simulink model "q_bb01_pos"  (R2021b)
settings: Solver=ode4  StartTime=0.0  StopTime=inf  FixedStep=0.002  RelTol=1e-3  AbsTol=1e-6  EnableMultiTasking=on
values from neighbouring files (symbols this model uses):
  K_AMP = 1    [setup_srv02_exp04_bb01.m]
  K_BS = - L_beam / 10    [config_bb01.m]    (also in setup_srv02_exp04_bb01.m = 2 * K_BS)
  Kc = wn^2 / (Tp*K_bb*z*wf)    [d_bb01_pd.m]    (also in setup_srv02_exp04_bb01.m = 0)
  kp = (wn^2/K)*tau    [d_pv_design.m]    (also in setup_srv02_exp04_bb01.m = 0)
  kv = (-1+2*zeta*wn*tau)/K    [d_pv_design.m]    (also in setup_srv02_exp04_bb01.m = 0)
  THETA_MAX = 56.0 * K_D2R    [config_bb01.m]
  THETA_MIN = - 56.0 * K_D2R    [config_bb01.m]
  THETA_OFF = - 56.0 * K_D2R    [config_bb01.m]
  VMAX_DAC = 10    [setup_srv02_exp04_bb01.m]
  wcf = 2 * pi * 50.0    (= 314.159265359)    [setup_srv02_exp04_bb01.m]
  wf = 2 * pi * 2.5    (= 15.7079632679)    [d_bb01_pd.m]    (also in setup_srv02_exp04_bb01.m = 6.28318530718)
  z = wn*wf/(-wn+wf*wn*Tp+2*wf*zeta)    [d_bb01_pd.m]    (also in setup_srv02_exp04_bb01.m = 1)
  zetaf = 0.9    [setup_srv02_exp04_bb01.m]
undefined symbols (not defined in the file or in its folder): HIL, K_ENC, qc_get_step_size, VMAX_AMP
libraries: simulink x6, quarc_library x6, simulink_extras x1
settings Model: SimulationMode=external  ExtModeTrigDuration=25000  Creator=MLevis  LastModifiedBy=Dell
settings SolverCC: AutoScaleAbsTol=off  AlgebraicLoopSolver=TrustRegion  PositivePriorityOrder=on
settings DataIOCC: SaveFormat=Array  SignalLoggingSaveFormat=ModelDataLogs  ReturnWorkspaceOutputs=off
settings OptimizationCC: BlockReduction=off  BooleanDataType=off  OptimizeBlockIOStorage=off  BufferReuse=off  ExpressionFolding=off  ExpressionDepthLimit=2147483647  LocalBlockOutputs=off  InitFltsAndDblsToZero=on
settings DebuggingCC: SaveWithParameterizedLinksMsg=none  UnderspecifiedInitializationDetection=Classic  MergeDetectMultiDrivingBlocksExec=none  SignalResolutionControl=TryResolveAllWithWarning  MultiTaskDSMMsg=warning  MultiTaskCondExecSysMsg=none  FcnCallInpInsideContextMsg=warning  StateNameClashWarn=warning  SFUnexpectedBacktrackingDiag=warning  SFNoUnconditionalDefaultTransitionDiag=warning  SFExecutionAtInitializationDiag=none  SFMachineParentedDataDiag=warning  ArithmeticOperatorsInVariantConditions=warning
settings HardwareCC: TargetHWDeviceType=32-bit Generic
settings ModelReferenceCC: PropagateSignalLabelsOutOfModel=off
settings RTWCC: Description=QUARC Win64 Target Using Toolchain  SystemTargetFile=quarc_win64.tlc  TemplateMakefile=quarc_default_tmf  Toolchain=QUARC win64 | nmake (64-bit Windows)  BuildConfiguration=Faster Runs
settings CodeAppCC: StateflowObjectComments=on
settings STFCustomTargetCC: ConcurrentExecutionCompliant=on  UseToolchainInfoCompliant=on  SystemTargetFile=quarc_win64.tlc
settings GRTTargetCC: TargetLangStandard=C89/C90 (ANSI)  ParMdlRefBuildCompliant=off  CompOptLevelCompliant=off  CombineOutputUpdateFcns=off  MatFileLogging=off  CPPClassGenCompliant=off  GRTInterface=on  ExtMode=on  ExtModeMexFile=quarc_comm
settings ConfigComp: CovMetricSettings=dw  CovSaveCumulativeToWorkspaceVar=on  CovSaveSingleToWorkspaceVar=on

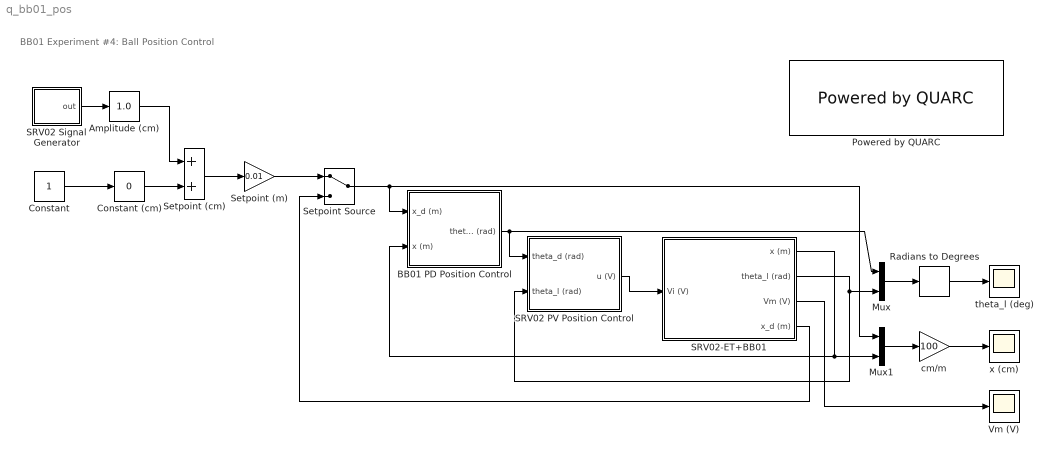
== system q_bb01_pos ==
  note: BB01 Experiment #4: Ball Position Control
  Amplitude (cm) : simulink/Math Operations/Slider Gain  gain=1.0  low=-10  high=10
  BB01 PD Position Control : Subsystem
  "Constant " : Constant
  Constant (cm) : simulink/Math Operations/Slider Gain  gain=0  low=-20  high=20
  Mux : Mux  Inputs=2
  Mux1 : Mux  Inputs=2
  Powered by QUARC : quarc_library/Logos/Powered by QUARC
  Radians to Degrees : simulink_extras/Transformations/Radians to Degrees
  SRV02 PV Position Control : Subsystem
  SRV02 Signal Generator : Subsystem  mask(QET Signal Generator){sig_type=square, a=2, f=0.4}
      mask prompts: sig_type "Signal Type"; a "Amplitude"; f "Frequency (Hz)"
      mask help: Generates a square, triangular, or sinusoidal waveform of a specified amplitude and frequency.
      mask Help: Choose the type of signal to be generated from the drop-down "Signal Type" box. Enter the amplitude and the frequency desired for the signal. Note: frequency is in Hertz.
      mask TypeOptions sig_type: square | triangle | sine
      mask Display: plot([0 1 1 2 2 3 4 5 6], [-1 -1 1 1 -1 -1 1 -1 -1])
  SRV02-ET+BB01 : Subsystem
  Setpoint Source : ManualSwitch
  Setpoint (cm) : Sum
  Setpoint (m) : Gain  Gain=0.01
  Vm (V) : Scope
  cm/m : Gain  Gain=100
  theta_l (deg) : Scope
  x (cm) : Scope
  wires:
  SRV02-ET+BB01/2(theta_l (rad)) -> Mux/2, SRV02 PV Position Control/2(theta_l (rad))
  SRV02 Signal Generator/1(out) -> Amplitude (cm)/1
  SRV02-ET+BB01/1(x (m)) -> Mux1/2, BB01 PD Position Control/2(x (m))
  Constant (cm)/1 -> Setpoint (cm)/2
  "Constant "/1 -> Constant (cm)/1
  Amplitude (cm)/1 -> Setpoint (cm)/1
  Radians to Degrees/1 -> theta_l (deg)/1
  Mux/1 -> Radians to Degrees/1
  Mux1/1 -> cm/m/1
  cm/m/1 -> x (cm)/1
  SRV02-ET+BB01/3(Vm (V)) -> Vm (V)/1
  SRV02 PV Position Control/1(u (V)) -> SRV02-ET+BB01/1(Vi (V))
  Setpoint (cm)/1 -> Setpoint (m)/1
  Setpoint (m)/1 -> Setpoint Source/1
  Setpoint Source/1 -> Mux1/1, BB01 PD Position Control/1(x_d (m))
  SRV02-ET+BB01/4(x_d (m)) -> Setpoint Source/2
  BB01 PD Position Control/1(theta_d (rad)) -> SRV02 PV Position Control/1(theta_d (rad)), Mux/1

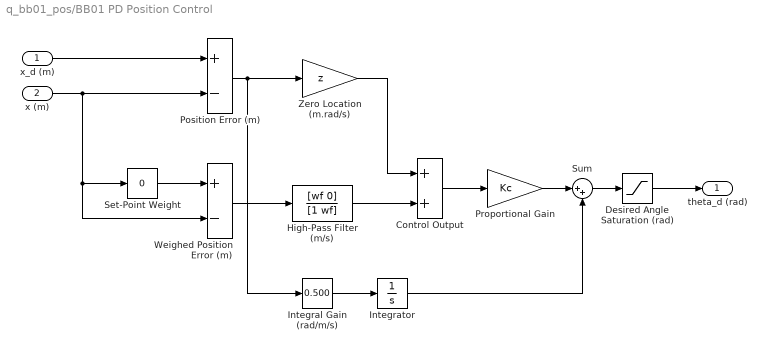
== system q_bb01_pos/BB01 PD Position Control ==
  x_d (m) : Inport
  x (m) : Inport  Port=2
  Control Output : Sum
  Desired Angle Saturation (rad) : Saturate  UpperLimit=THETA_MAX  LowerLimit=THETA_MIN
  High-Pass Filter (m/s) : TransferFcn  Numerator=[wf 0]  Denominator=[1 wf]
  Integral Gain (rad/m/s) : simulink/Math Operations/Slider Gain  gain=0.500  low=0  high=5
  Integrator : Integrator  LimitOutput=on  UpperSaturationLimit=THETA_MAX  LowerSaturationLimit=THETA_MIN
  Position Error (m) : Sum  Inputs=+-
  "Proportional Gain " : Gain  Gain=Kc
  Set-Point Weight : simulink/Math Operations/Slider Gain  gain=0  low=0  high=1
  Sum : Sum  Inputs=|++
  Weighed Position Error (m) : Sum  Inputs=+-
  Zero Location (m.rad/s) : Gain  Gain=z
  theta_d (rad) : Outport
  wires:
  Sum/1 -> Desired Angle Saturation (rad)/1
  "Proportional Gain "/1 -> Sum/1
  Desired Angle Saturation (rad)/1 -> theta_d (rad)/1
  Integral Gain (rad/m/s)/1 -> Integrator/1
  High-Pass Filter (m/s)/1 -> Control Output/2
  Zero Location (m.rad/s)/1 -> Control Output/1
  Control Output/1 -> "Proportional Gain "/1
  Weighed Position Error (m)/1 -> High-Pass Filter (m/s)/1
  Set-Point Weight/1 -> Weighed Position Error (m)/1
  x_d (m)/1 -> Position Error (m)/1
  x (m)/1 -> Weighed Position Error (m)/2, Set-Point Weight/1, Position Error (m)/2
  Position Error (m)/1 -> Integral Gain (rad/m/s)/1, Zero Location (m.rad/s)/1
  Integrator/1 -> Sum/2

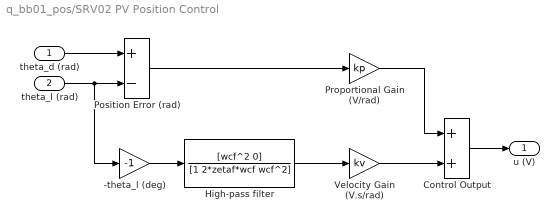
== system q_bb01_pos/SRV02 PV Position Control ==
  theta_d (rad) : Inport
  theta_l (rad) : Inport  Port=2
  -theta_l (deg) : Gain  Gain=-1
  Control Output : Sum
  High-pass filter : TransferFcn  Numerator=[wcf^2 0]  Denominator=[1 2*zetaf*wcf wcf^2]
  Position Error (rad) : Sum  Inputs=+-
  Proportional Gain (V/rad) : Gain  Gain=kp
  Velocity Gain (V.s/rad) : Gain  Gain=kv
  u (V) : Outport
  wires:
  Velocity Gain (V.s/rad)/1 -> Control Output/2
  -theta_l (deg)/1 -> High-pass filter/1
  Position Error (rad)/1 -> Proportional Gain (V/rad)/1
  theta_l (rad)/1 -> -theta_l (deg)/1, Position Error (rad)/2
  Control Output/1 -> u (V)/1
  theta_d (rad)/1 -> Position Error (rad)/1
  Proportional Gain (V/rad)/1 -> Control Output/1
  High-pass filter/1 -> Velocity Gain (V.s/rad)/1

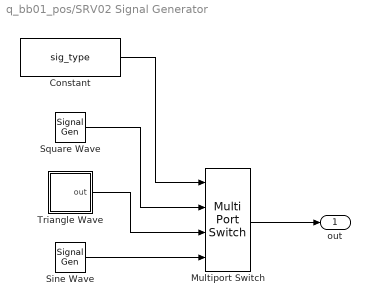
== system q_bb01_pos/SRV02 Signal Generator ==
  Constant : Constant  Value=sig_type
  Multiport Switch : MultiPortSwitch
  Sine Wave : SignalGenerator  Amplitude=a  Frequency=f
  Square Wave : SignalGenerator  WaveForm=square  Amplitude=a  Frequency=f
  Triangle Wave : Subsystem
  out : Outport
  wires:
  Constant/1 -> Multiport Switch/1
  Multiport Switch/1 -> out/1
  Sine Wave/1 -> Multiport Switch/4
  Triangle Wave/1(out) -> Multiport Switch/3
  Square Wave/1 -> Multiport Switch/2

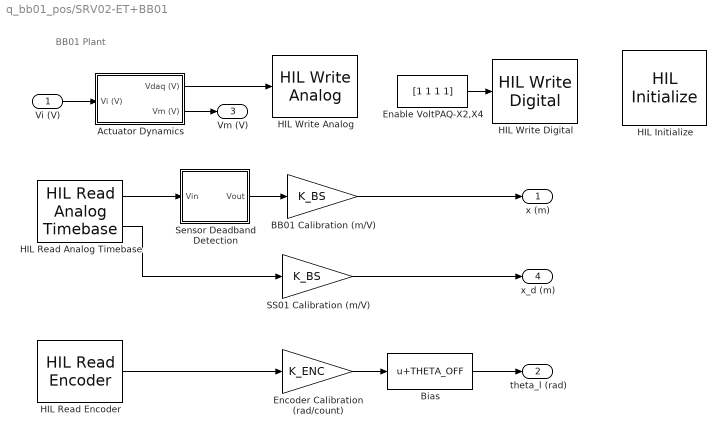
== system q_bb01_pos/SRV02-ET+BB01 ==
  note: BB01 Plant
  Vi (V) : Inport
  Actuator Dynamics : Subsystem
  BB01 Calibration (m/V) : Gain  Gain=K_BS  SaturateOnIntegerOverflow=on  OutDataTypeStr=Inherit: Same as input  ParamDataTypeStr=Inherit: Same as input
  Bias : Bias  Bias=THETA_OFF
  Enable VoltPAQ-X2,X4 : Constant  Value=[1 1 1 1]
  Encoder Calibration (rad/count) : Gain  Gain=K_ENC  SaturateOnIntegerOverflow=on  OutDataTypeStr=Inherit: Same as input  ParamDataTypeStr=Inherit: Same as input
  HIL Initialize : quarc_library/Data Acquisition/Generic/Configuration/HIL Initialize  object_name=HIL-1  board_type=q8_usb  board_number=0  board_options=update_rate=normal  exclusive=off  active=off  hardware_clocks=[0:2]  clock_modes=[]  initial_clock_frequencies=[]  set_clock_params_at_start=off  set_clock_params_at_switch_in=off  set_clock_frequencies_at_start=off  set_clock_frequencies_at_switch_in=off  analog_input_channels=[0:7]  analog_input_configurations=[]  analog_input_maximums=10  analog_input_minimums=-10  set_analog_input_params_at_start=on  set_analog_input_params_at_switch_in=off  analog_output_channels=[0:7]  analog_output_maximums=10  analog_output_minimums=-10  initial_analog_outputs=[0]  final_analog_outputs=[0]  watchdog_analog_outputs=0  set_analog_output_params_at_start=on  set_analog_output_params_at_switch_in=off  set_analog_outputs_at_start=on  set_analog_outputs_at_switch_in=off  set_analog_outputs_at_terminate=on  set_analog_outputs_at_switch_out=off  set_analog_outputs_on_watchdog=off  digital_input_channels=[]  digital_output_channels=[0:7]  digital_output_configuration=[]  initial_digital_outputs=[0]  final_digital_outputs=[0]  watchdog_digital_outputs=[0]  set_digital_output_params_at_start=off  set_digital_output_params_at_switch_in=off  set_digital_outputs_at_start=on  set_digital_outputs_at_switch_in=off  set_digital_outputs_at_terminate=on  set_digital_outputs_at_switch_out=off  set_digital_outputs_on_watchdog=off  encoder_channels=[0:7]  quadrature=[4]  encoder_filter_frequency=[]  initial_encoder_counts=[0]  set_encoder_params_at_start=on  set_encoder_params_at_switch_in=off  set_encoder_counts_at_start=on  set_encoder_counts_at_switch_in=off  pwm_channels=[0:7]  pwm_modes=0  pwm_frequency=99.532799999999995e6/4095  pwm_configuration=[0]  pwm_alignment=[0]  pwm_polarity=[1]  pwm_leading_deadband=[0]  pwm_trailing_deadband=[0]  initial_pwm_outputs=[0]  final_pwm_outputs=[0]  watchdog_pwm_outputs=[0]  set_pwm_params_at_start=on  set_pwm_params_at_switch_in=off  set_pwm_outputs_at_start=on  set_pwm_outputs_at_switch_in=off  set_pwm_outputs_at_terminate=on  set_pwm_outputs_at_switch_out=off  set_pwm_outputs_on_watchdog=off  other_output_channels=[]  initial_other_outputs=[]  final_other_outputs=[]  watchdog_other_outputs=[]  set_other_outputs_at_start=off  set_other_outputs_at_switch_in=off  set_other_outputs_at_terminate=off  set_other_outputs_at_switch_out=off  set_other_outputs_on_watchdog=off
  HIL Read Analog Timebase : quarc_library/Data Acquisition/Generic/Timebases/HIL Read Analog Timebase  Tag=unassigned  object_name=HIL-1  channels=[0:1]  clock=0  active=on  vector_output=off  overflow_mode=Error on overflow  samples_in_buffer=max(ceil(1/qc_get_step_size), 1)
      settings: AttributesFormatString=(%<object_name>)  SourceProductName=QUARC Targets
  HIL Read Encoder : quarc_library/Data Acquisition/Generic/Immediate I//O/HIL Read Encoder  Tag=unassigned  object_name=HIL-1  channels=0  sample_time=qc_get_step_size  active=on  vector_output=off  data_type_mode=Inherit via back propagation  data_type=double
  HIL Write Analog : quarc_library/Data Acquisition/Generic/Immediate I//O/HIL Write Analog  Tag=unassigned  object_name=HIL-1  channels=0  sample_time=-1  active=off  vector_input=off
  HIL Write Digital : quarc_library/Data Acquisition/Generic/Immediate I//O/HIL Write Digital  object_name=HIL-1  channels=[0:3]  sample_time=-1  active=off  vector_input=on
      settings: SourceProductName=QUARC Targets
  SS01 Calibration (m/V) : Gain  Gain=K_BS  SaturateOnIntegerOverflow=on  OutDataTypeStr=Inherit: Same as input  ParamDataTypeStr=Inherit: Same as input
  Sensor Deadband Detection : Subsystem
  x (m) : Outport  InitialOutput=0
  theta_l (rad) : Outport  Port=2  InitialOutput=0
  Vm (V) : Outport  Port=3  InitialOutput=0
  x_d (m) : Outport  Port=4  InitialOutput=0
  wires:
  HIL Read Encoder/1 -> Encoder Calibration (rad/count)/1
  Actuator Dynamics/2(Vm (V)) -> Vm (V)/1
  Actuator Dynamics/1(Vdaq (V)) -> HIL Write Analog/1
  Vi (V)/1 -> Actuator Dynamics/1(Vi (V))
  Encoder Calibration (rad/count)/1 -> Bias/1
  Bias/1 -> theta_l (rad)/1
  BB01 Calibration (m/V)/1 -> x (m)/1
  Sensor Deadband Detection/1(Vout) -> BB01 Calibration (m/V)/1
  HIL Read Analog Timebase/2 -> SS01 Calibration (m/V)/1
  SS01 Calibration (m/V)/1 -> x_d (m)/1
  HIL Read Analog Timebase/1 -> Sensor Deadband Detection/1(Vin)
  Enable VoltPAQ-X2,X4/1 -> HIL Write Digital/1

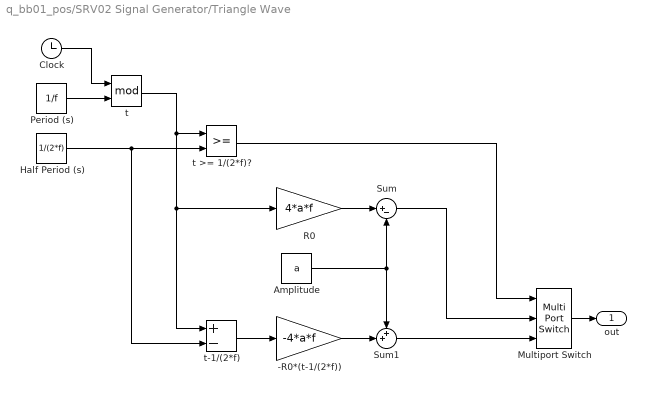
== system q_bb01_pos/SRV02 Signal Generator/Triangle Wave ==
  -R0*(t-1/(2*f)) : Gain  Gain=-4*a*f
  Amplitude : Constant  Value=a
  Clock : Clock
  Half Period (s) : Constant  Value=1/(2*f)
  Multiport Switch : MultiPortSwitch  DataPortOrder=Zero-based contiguous  Inputs=2  zeroidx=on
  Period (s) : Constant  Value=1/f
  R0 : Gain  Gain=4*a*f
  Sum : Sum  Inputs=|+-
  Sum1 : Sum  Inputs=++|
  t : Math  Operator=mod  SignedPower=on  SaturateOnIntegerOverflow=on
  t >= 1/(2*f)? : RelationalOperator  OutDataTypeStr=boolean  RndMeth=Nearest
  t-1/(2*f) : Sum  Inputs=+-
  out : Outport
  wires:
  Multiport Switch/1 -> out/1
  Clock/1 -> t/1
  Period (s)/1 -> t/2
  t/1 -> t >= 1/(2*f)?/1, R0/1, t-1/(2*f)/1
  Half Period (s)/1 -> t >= 1/(2*f)?/2, t-1/(2*f)/2
  t-1/(2*f)/1 -> -R0*(t-1/(2*f))/1
  R0/1 -> Sum/1
  Amplitude/1 -> Sum/2, Sum1/1
  -R0*(t-1/(2*f))/1 -> Sum1/2
  t >= 1/(2*f)?/1 -> Multiport Switch/1
  Sum/1 -> Multiport Switch/2
  Sum1/1 -> Multiport Switch/3

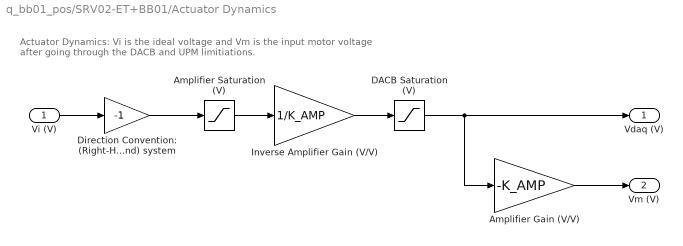
== system q_bb01_pos/SRV02-ET+BB01/Actuator Dynamics ==
  note: Actuator Dynamics: Vi is the ideal voltage and Vm is the
      | input motor voltage after going through the DACB and UPM limitiations.
  Vi (V) : Inport
  Amplifier Gain (V/V) : Gain  Gain=-K_AMP
  Amplifier Saturation (V) : Saturate  UpperLimit=VMAX_AMP  LowerLimit=-VMAX_AMP
  DACB Saturation (V) : Saturate  UpperLimit=VMAX_DAC  LowerLimit=-VMAX_DAC
  Direction Convention: (Right-Hand) system : Gain  Gain=-1  SaturateOnIntegerOverflow=on  OutDataTypeStr=Inherit: Same as input  ParamDataTypeStr=Inherit: Same as input
  Inverse Amplifier Gain (V/V) : Gain  Gain=1/K_AMP
  Vdaq (V) : Outport
  Vm (V) : Outport  Port=2
  wires:
  Direction Convention: (Right-Hand) system/1 -> Amplifier Saturation (V)/1
  Amplifier Gain (V/V)/1 -> Vm (V)/1
  DACB Saturation (V)/1 -> Vdaq (V)/1, Amplifier Gain (V/V)/1
  Inverse Amplifier Gain (V/V)/1 -> DACB Saturation (V)/1
  Vi (V)/1 -> Direction Convention: (Right-Hand) system/1
  Amplifier Saturation (V)/1 -> Inverse Amplifier Gain (V/V)/1

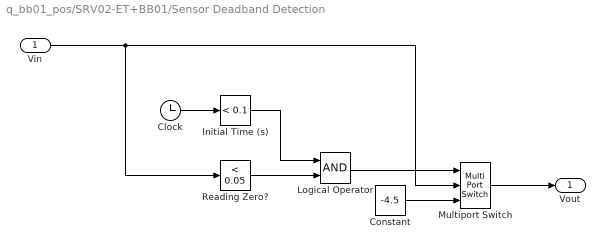
== system q_bb01_pos/SRV02-ET+BB01/Sensor Deadband Detection ==
  Vin : Inport
  Clock : Clock
  Constant : Constant  Value=-4.5
  Initial Time (s) : simulink/Logic and Bit Operations/Compare To Constant  relop=<  const=0.1  OutDataTypeStr=uint8  ZeroCross=off
  Logical Operator : Logic  AllPortsSameDT=off  OutDataTypeStr=boolean
  Multiport Switch : MultiPortSwitch  DataPortOrder=Zero-based contiguous  Inputs=2  zeroidx=on
  Reading Zero? : simulink/Logic and Bit Operations/Compare To Constant  relop=<  const=0.05  OutDataTypeStr=uint8  ZeroCross=off
  Vout : Outport
  wires:
  Clock/1 -> Initial Time (s)/1
  Vin/1 -> Reading Zero?/1, Multiport Switch/2
  Initial Time (s)/1 -> Logical Operator/1
  Reading Zero?/1 -> Logical Operator/2
  Logical Operator/1 -> Multiport Switch/1
  Constant/1 -> Multiport Switch/3
  Multiport Switch/1 -> Vout/1
